simulink model "tetheredKiteModel"  (R2019a)
settings: Solver=VariableStepAuto  StartTime=0.0  StopTime=20  RelTol=1e-3
undefined symbols (not defined in the file or in its folder): magnitude
libraries: angleBtw2Vecs_ul x5, accelerationCalculator_ul x5, vrlib x4
(part 1 of 2)
settings Model: Creator=jcreed2  LastModifiedBy=jcreed2
settings DataIOCC: SaveFormat=StructureWithTime

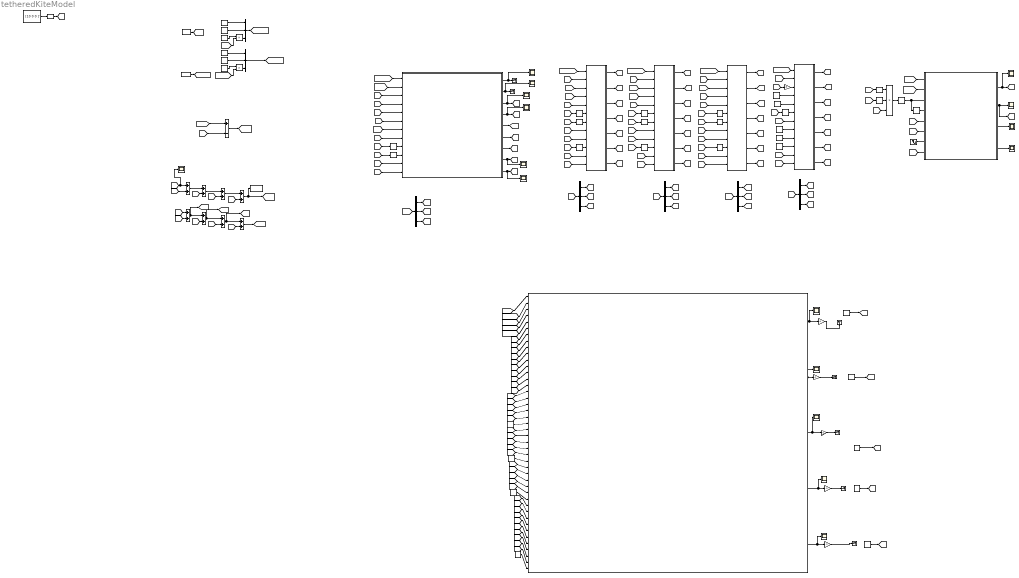
== system tetheredKiteModel ==
  note: ground position and vel.
  note: Tension Calculation
  note: Controller
  note: nodes 2-5
  note: Tether node at kite
  note: Gravity and Kite Force Calculation
  note: Kite Forces
  note: gravity force in the ground frame
  note: Force Gravity
  note: Env
  Add{,1..7} (8 alike) : Sum
  Constant : Constant  Value=[10 0 0 ]'
  Constant{1..2,5..6,10..12,15..17} (10 alike) : Constant  Value=0
  Constant13 : Constant  Value=[0,0,0]'
  Constant14 : Constant  Value=[0,0,0]'
  Constant{18..22} (5 alike) : Constant  Value=900
  Constant3 : Constant  Value=-9.81
  Constant4 : Constant  Value=20 + .5*1000*200*pi*.0005*.0005
  Constant7 : Constant  Value=-9.81
  Constant8 : Constant  Value=200
  Constant9 : Constant  Value=1000*200*pi*.0005*.0005
  Cos13 : Trigonometry  Operator=cos
  Cos14 : Trigonometry  Operator=cos
  Demux{,1..4} (5 alike) : Demux  Outputs=3
  Divide : Product  Inputs=**
  Divide1 : Product  Inputs=**
  Divide28 : Product  Inputs=***
  MATLAB Function2 : MATLAB Function  TreatAsAtomicUnit=on
  Memory{,1..13} (14 alike) : Memory
  Minus : Sum  Inputs=+-
  Multiply : Gain  Gain=.5
  Multiply{1..5} (5 alike) : Gain  Gain=-1
  Reshape : Reshape  OutputDimensionality=Column vector (2-D)
  Scope{,1..12,14..16} (16 alike) : Scope
  Sine Wave : Sin  Amplitude=60  Frequency=1/20  SampleTime=0
  Subsystem : Subsystem  mask{ky1=.1, ky=.01, kydot=.1, kalpha=0.001, rMin=-0.3491, rMax=0.3491, aMin=-0.0873, aMax=0.0873}
      mask prompts: rMin "roll min"; rMax "roll max"; aMin "aoaBar min"; aMax "aoaBar max"
  Terminator{,1..6} (7 alike) : Terminator
  To Workspace : ToWorkspace  VariableName=kitePos  SaveFormat=Timeseries  SampleTime=-1
  Vector Concatenate : Concatenate  NumInputs=3
  Vector Concatenate1 : Concatenate  NumInputs=3
  node2 : Subsystem  mask{rho=1.23, cD=1.2, lq=200, d=.001}
      mask prompts: lq "linkLength"; d "tether diameter"
  node3 : Subsystem  mask{rho=1.23, cD=1.2, lq=200, d=.001}
      mask prompts: lq "linkLength"; d "tether diameter"
  node4 : Subsystem  mask{rho=1.23, cD=1.2, lq=200, d=.001}
      mask prompts: lq "linkLength"; d "tether diameter"
  "node5 " : Subsystem  mask{rho=1.23, cD=1.2, lq=200, d=.001}
      mask prompts: lq "linkLength"; d "tether diameter"
  "tether node one (kite end of the tether) " : Subsystem  mask{cLA=4.4, S=25, rho=1.23, cD=1.2, lq=200, d=.001, cdO=.02, kO=.1}
      mask prompts: lq "linkLength"; d "tetherDiameter"; cdO "cd0"; kO "k0"
  wires:
  Constant/1 -> Reshape/1
  Reshape/1 -> [vWind]
  Constant1/1 -> Vector Concatenate/1
  Constant2/1 -> Vector Concatenate/2
  Constant3/1 -> Divide/1
  Constant4/1 -> [kiteMass]
  Divide/1 -> Vector Concatenate/3
  Vector Concatenate/1 -> [FGravKite]
  Divide1/1 -> Vector Concatenate1/3
  Constant6/1 -> Vector Concatenate1/2
  Constant5/1 -> Vector Concatenate1/1
  [tetherNodeMass] -> Divide1/2
  Constant7/1 -> Divide1/1
  Vector Concatenate1/1 -> [FGravTetherNodes]
  [FGravKite] -> "tether node one (kite end of the tether) "/1(kiteGrav)
  Constant9/1 -> [tetherNodeMass]
  [kiteMass] -> Divide/2
  [vWind] -> Minus/2
  [link1Vel] -> Minus/1  "kiteVel"
  Minus/1 -> [vRelGnd]  "vRel"
  [vRelGnd] -> Subsystem/2("vRelGnd ")
  Subsystem/1(roll) -> Scope/1, [roll]
  Subsystem/2(alpha) -> Scope3/1, [alpha]
  "tether node one (kite end of the tether) "/2("fDrag ") -> Scope12/1, Terminator/1  "fDrag"
  "tether node one (kite end of the tether) "/1("fLift ") -> Scope11/1, Terminator1/1  "fLift"
  "tether node one (kite end of the tether) "/5(fExt1) -> [fExtKite]  "fExt1"
  "tether node one (kite end of the tether) "/3(theta1) -> Scope9/1, [theta1]
  "tether node one (kite end of the tether) "/4(phi1) -> Scope10/1, [phi1]
  [theta1] -> Subsystem/5(theta)
  [phi1] -> Subsystem/6(phi)
  [vRelGnd] -> "tether node one (kite end of the tether) "/2(vRelGnd)
  [alpha] -> "tether node one (kite end of the tether) "/4(alpha)
  [roll] -> "tether node one (kite end of the tether) "/3(roll)
  [vWind] -> "tether node one (kite end of the tether) "/5(vWind)
  "tether node one (kite end of the tether) "/6("r1 ") -> [r1]
  "tether node one (kite end of the tether) "/7(r1Dot) -> [r1Dot]  "r1Dot"
  [fExtKite] -> Demux/1
  Demux/1 -> [fx1]
  Demux/2 -> [fy1]
  Demux/3 -> [fz1]
  [tetherNodeMass] -> MATLAB Function2/2(m2)
  [kiteMass] -> MATLAB Function2/1(m1)
  [tetherNodeMass] -> MATLAB Function2/3(m3)
  [tetherNodeMass] -> MATLAB Function2/4(m4)
  [tetherNodeMass] -> MATLAB Function2/5(m5)
  [phi1] -> MATLAB Function2/11(p1)
  [theta1] -> MATLAB Function2/6(t1)
  [fx1] -> MATLAB Function2/16(fx1)
  [fz1] -> MATLAB Function2/28(fz1)
  [fy1] -> MATLAB Function2/22(fy1)
  "tether node one (kite end of the tether) "/8(p1d) -> Scope14/1, [p1d]
  [p1d] -> MATLAB Function2/39(p1d)
  [t1d] -> MATLAB Function2/34(t1d)
  Constant8/1 -> MATLAB Function2/44(L)
  MATLAB Function2/3(ten3) -> Scope6/1, Multiply3/1  "ten3"
  MATLAB Function2/4(ten4) -> Scope7/1, Multiply4/1  "ten4"
  MATLAB Function2/5(ten5) -> Scope8/1, Multiply5/1  "ten5"
  [ten1] -> Memory1/1
  [FGravTetherNodes] -> node2/1(nodeGrav)
  [vWind] -> node2/2(vWind)
  [ten2] -> Memory3/1
  [ten1] -> Memory4/1
  [ten2] -> Memory2/1
  [theta1] -> node2/11(thetaq01)
  [phi1] -> node2/12(phiq01)
  [ten3] -> Memory7/1
  node2/5(rqDot) -> [r2Dot]  "r2Dot"
  node2/4("rq ") -> [r2]
  node2/3(fExtq) -> [fExt2]  "fExt2"
  node2/6(pqd) -> [p2d]
  node2/7(tqd) -> [t2d]
  node2/2(phiq) -> [phi2]
  node2/1(thetaq) -> [theta2]
  [fExt2] -> "tether node one (kite end of the tether) "/8(Fext2)
  [theta2] -> "tether node one (kite end of the tether) "/11("theta2 ")
  [phi2] -> "tether node one (kite end of the tether) "/12(phi2)
  Demux1/3 -> [fz2]
  [fExt2] -> Demux1/1
  Demux1/1 -> [fx2]
  Demux1/2 -> [fy2]
  [fx2] -> MATLAB Function2/17(fx2)
  [fy2] -> MATLAB Function2/23(fy2)
  [fz2] -> MATLAB Function2/29(fz2)
  [phi2] -> MATLAB Function2/12(p2)
  [theta2] -> MATLAB Function2/7(t2)
  [p2d] -> MATLAB Function2/40(p2d)
  [t2d] -> MATLAB Function2/35(t2d)
  [FGravTetherNodes] -> node3/1(nodeGrav)
  node3/1(thetaq) -> [theta3]
  node3/2(phiq) -> [phi3]
  node3/5(rqDot) -> [r3Dot]  "r3Dot"
  node3/7(tqd) -> [t3d]
  [ten3] -> Memory5/1
  [vWind] -> node3/2(vWind)
  [theta2] -> node3/11(thetaq01)
  [ten4] -> Memory8/1
  node3/6(pqd) -> [p3d]
  [ten2] -> Memory6/1
  node3/3(fExtq) -> [fExt3]  "fExt3"
  [phi2] -> node3/12(phiq01)
  node3/4("rq ") -> [r3]
  [theta3] -> node2/8("thetaq1 ")
  [phi3] -> node2/9(phiq1)
  [fExt3] -> node2/5(Fextq1)
  [fExt3] -> Demux2/1
  Demux2/2 -> [fy3]
  Demux2/1 -> [fx3]
  Demux2/3 -> [fz3]
  [theta3] -> MATLAB Function2/8(t3)
  [phi3] -> MATLAB Function2/13(p3)
  [fx3] -> MATLAB Function2/18(fx3)
  [fy3] -> MATLAB Function2/24(fy3)
  [fz3] -> MATLAB Function2/30(fz3)
  [t3d] -> MATLAB Function2/36(t3d)
  [p3d] -> MATLAB Function2/41(p3d)
  [p4d] -> MATLAB Function2/42(p4d)
  [p5d] -> MATLAB Function2/43(p5d)
  [t5d] -> MATLAB Function2/38(t5d)
  [t4d] -> MATLAB Function2/37(t4d)
  [fz4] -> MATLAB Function2/31(fz4)
  [fz5] -> MATLAB Function2/32(fz5)
  [fy4] -> MATLAB Function2/25(fy4)
  [fy5] -> MATLAB Function2/26(fy5)
  [fx5] -> MATLAB Function2/20(fx5)
  [fx4] -> MATLAB Function2/19(fx4)
  [phi5] -> MATLAB Function2/15(p5)
  [phi4] -> MATLAB Function2/14(p4)
  [theta4] -> MATLAB Function2/9(t4)
  [theta5] -> MATLAB Function2/10(t5)
  Demux3/2 -> [fy4]
  Demux3/3 -> [fz4]
  Demux3/1 -> [fx4]
  node4/4("rq ") -> [r4]
  [ten3] -> Memory10/1
  [phi3] -> node4/12(phiq01)
  node4/3(fExtq) -> [fExt4]  "fExt4"
  [fExt4] -> Demux3/1
  [ten4] -> Memory9/1
  [vWind] -> node4/2(vWind)
  node4/7(tqd) -> [t4d]
  node4/5(rqDot) -> [r4Dot]  "r4Dot"
  [ten5] -> Memory11/1
  [theta3] -> node4/11(thetaq01)
  node4/1(thetaq) -> [theta4]
  node4/6(pqd) -> [p4d]
  node4/2(phiq) -> [phi4]
  [FGravTetherNodes] -> node4/1(nodeGrav)
  [theta4] -> node3/8("thetaq1 ")
  [phi4] -> node3/9(phiq1)
  [fExt4] -> node3/5(Fextq1)
  [fExt5] -> node4/5(Fextq1)
  [theta5] -> node4/8("thetaq1 ")
  [phi5] -> node4/9(phiq1)
  Constant11/1 -> "node5 "/9(phiq1)
  Constant12/1 -> "node5 "/8("thetaq1 ")
  "node5 "/2(phiq) -> [phi5]
  Constant10/1 -> "node5 "/10(tenq1)
  "node5 "/1(thetaq) -> [theta5]
  "node5 "/5(rqDot) -> [r5Dot]  "r5Dot"
  "node5 "/7(tqd) -> [t5d]
  [ten4] -> "node5 "/7(tenq01)
  [theta4] -> "node5 "/11(thetaq01)
  [ten5] -> Memory12/1
  "node5 "/3(fExtq) -> [fExt5]  "fExt5"
  [FGravTetherNodes] -> "node5 "/1(nodeGrav)
  "node5 "/6(pqd) -> [p5d]
  "node5 "/4("rq ") -> [r5]
  [vWind] -> "node5 "/2(vWind)
  [phi4] -> "node5 "/12(phiq01)
  [r5] -> Scope2/1, Add/1  "node5Pos"
  [r4] -> Add/2
  Add/1 -> Add1/1  "node4Pos"
  Add1/1 -> Add2/1  "node3Pos"
  [r3] -> Add1/2
  Constant13/1 -> "node5 "/4(linkQ1VelGnd)
  [fExt5] -> Demux4/1
  Demux4/1 -> [fx5]
  Demux4/2 -> [fy5]
  Demux4/3 -> [fz5]
  [r2] -> Add2/2
  Add2/1 -> Add3/1  "node2Pos"
  [r1] -> Add3/2
  Add3/1 -> To Workspace/1, [kitePosGnd]  "kitePosGnd"
  [kitePosGnd] -> Subsystem/1("kitePosGnd ")
  [r4Dot] -> Add4/2
  Add4/1 -> [link4Vel], Add5/1  "link4Vel"
  [r1Dot] -> Add7/2
  [r5Dot] -> Add4/1
  [r2Dot] -> Add6/2
  [r3Dot] -> Add5/2
  Add5/1 -> Add6/1, [link3Vel]  "link3Vel"
  Add7/1 -> [link1Vel]
  Add6/1 -> [link2Vel], Add7/1
  Multiply/1 -> "node5 "/3("linkQVelGnd ")
  [link2Vel] -> "tether node one (kite end of the tether) "/7(link2VelGnd)  "link2Vel"
  [link3Vel] -> node2/4(linkQ1VelGnd)
  [link2Vel] -> node2/3("linkQVelGnd ")
  [link1Vel] -> "tether node one (kite end of the tether) "/6("kiteVelGnd ")
  [link3Vel] -> node3/3("linkQVelGnd ")
  [link4Vel] -> node3/4(linkQ1VelGnd)
  [link4Vel] -> node4/3("linkQVelGnd ")
  [r5Dot] -> node4/4(linkQ1VelGnd)
  Sine Wave/1 -> Subsystem/7("sineWave ")
  Memory/1 -> Subsystem/4("Tk01 ")
  Divide28/1 -> Memory13/1
  Cos13/1 -> Divide28/1
  [ten1] -> Divide28/3
  [theta1] -> Cos13/1
  Cos14/1 -> Divide28/2
  [phi1] -> Cos14/1
  Constant14/1 -> "node5 "/5(Fextq1)
  Constant15/1 -> MATLAB Function2/21(fx6)
  Constant17/1 -> MATLAB Function2/33(fz6)
  Constant16/1 -> MATLAB Function2/27(fy6)
  Memory1/1 -> "tether node one (kite end of the tether) "/9("ten1 ")
  Memory2/1 -> "tether node one (kite end of the tether) "/10(ten2)
  Memory4/1 -> node2/7(tenq01)
  Memory3/1 -> node2/6("tenq ")
  Memory5/1 -> node3/6("tenq ")
  Memory6/1 -> node3/7(tenq01)
  Memory7/1 -> node2/10(tenq1)
  Memory8/1 -> node3/10(tenq1)
  Memory9/1 -> node4/6("tenq ")
  Memory10/1 -> node4/7(tenq01)
  Memory11/1 -> node4/10(tenq1)
  Memory12/1 -> "node5 "/6("tenq ")
  Memory13/1 -> Memory/1, Subsystem/3("Tc ")
  [link1Vel] -> Subsystem/8("kiteVelGnd ")
  Subsystem/3(error) -> Scope1/1
  [r5Dot] -> Multiply/1
  MATLAB Function2/1(ten1) -> Scope4/1, Multiply1/1  "ten"
  MATLAB Function2/2(ten2) -> Scope5/1, Multiply2/1  "ten2"
  "tether node one (kite end of the tether) "/9(t1d) -> Scope15/1, [t1d]
  Multiply1/1 -> Terminator2/1
  Multiply3/1 -> Terminator4/1
  Multiply5/1 -> Terminator6/1
  Subsystem/4(tenError) -> Scope16/1
  Constant18/1 -> [ten1]
  Constant19/1 -> [ten2]
  Multiply2/1 -> Terminator3/1
  Constant20/1 -> [ten3]
  Constant21/1 -> [ten4]
  Multiply4/1 -> Terminator5/1
  Constant22/1 -> [ten5]

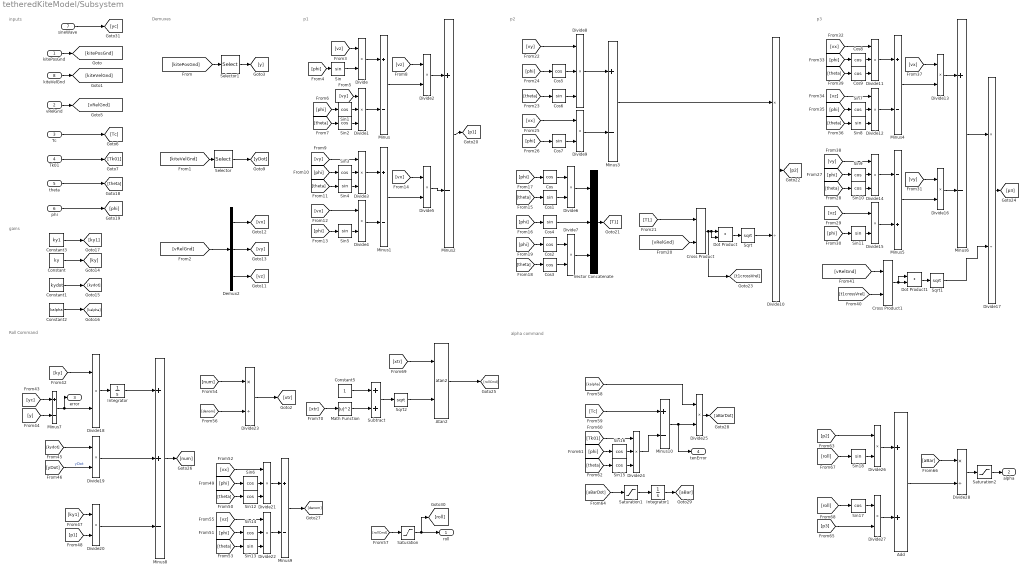
== system tetheredKiteModel/Subsystem ==
  note: alpha command
  note: Roll Command
  note: p2
  note: p1
  note: gains
  note: Demuxes
  note: inputs
  note: p3
  "kitePosGnd " : Inport
  "vRelGnd " : Inport  Port=2
  "Tc " : Inport  Port=3
  "Tk01 " : Inport  Port=4
  theta : Inport  Port=5
  phi : Inport  Port=6
  "sineWave " : Inport  Port=7
  "kiteVelGnd " : Inport  Port=8
  Add : Sum
  Atan2 : Trigonometry  Operator=atan2
  Constant : Constant  Value=ky
  Constant1 : Constant  Value=kydot
  Constant2 : Constant  Value=kalpha
  Constant3 : Constant  Value=ky1
  Constant5 : Constant
  Cos{,2..3,5,8..9} (6 alike) : Trigonometry  Operator=cos
  Cos{1,4,6..7} (4 alike) : Trigonometry
  Cross Product : vrlib/Utilities/Cross Product
      settings: SourceProductName=Simulink
  Cross Product1 : vrlib/Utilities/Cross Product
      settings: SourceProductName=Simulink
  Demux2 : Demux  Outputs=3
  Divide{,2,4..7,9,13,15..16,18..20,25..27} (16 alike) : Product  Inputs=**
  Divide{1,3,8,11..12,14,21..22,24} (9 alike) : Product  Inputs=***
  Divide{10,17,23,28} (4 alike) : Product  Inputs=*/
  Dot Product : DotProduct  InputSameDT=on  OutDataTypeStr=Inherit: Inherit via internal rule
  Dot Product1 : DotProduct  InputSameDT=on  OutDataTypeStr=Inherit: Inherit via internal rule
  Integrator : Integrator
  Integrator1 : Integrator
  Math Function : Math  Operator=magnitude^2  SaturateOnIntegerOverflow=on
  Minus{,1..4,6..7,9..10} (9 alike) : Sum  Inputs=+-
  Minus5 : Sum  Inputs=-+
  Minus8 : Sum  Inputs=++-
  Saturation : Saturate  UpperLimit=rMax  LowerLimit=rMin
  Saturation1 : Saturate  UpperLimit=aMax  LowerLimit=aMin
  Saturation2 : Saturate  UpperLimit=0.0349*4  LowerLimit=0.0349
  Selector : Selector  InputPortWidth=3  IndexOptions=Index vector (dialog)  Indices=2  OutputSizes=1
  Selector1 : Selector  InputPortWidth=3  IndexOptions=Index vector (dialog)  Indices=2  OutputSizes=1
  Sin{,4..5,8,11,13,18} (7 alike) : Trigonometry
  Sin{1..3,6..7,9..10,12,14..17} (12 alike) : Trigonometry  Operator=cos
  Sqrt : Sqrt  SaturateOnIntegerOverflow=on
  Sqrt1 : Sqrt  SaturateOnIntegerOverflow=on
  Sqrt2 : Sqrt  SaturateOnIntegerOverflow=on
  Subtract : Sum
  Vector Concatenate : Concatenate  NumInputs=3
  roll : Outport
  alpha : Outport  Port=2
  error : Outport  Port=3
  tenError : Outport  Port=4
  wires:
  "kitePosGnd "/1 -> [kitePosGnd]
  "kiteVelGnd "/1 -> [kiteVelGnd]
  "vRelGnd "/1 -> [vRelGnd]
  "Tc "/1 -> [Tc]
  "Tk01 "/1 -> [Tk01]
  [kiteVelGnd] -> Selector/1
  Selector/1 -> [yDot]
  [vRelGnd] -> Demux2/1
  Demux2/1 -> [vx]
  Demux2/2 -> [vy]
  Demux2/3 -> [vz]
  Constant/1 -> [ky]
  Constant1/1 -> [kydot]
  Constant2/1 -> [kalpha]
  Constant3/1 -> [ky1]
  theta/1 -> [theta]
  phi/1 -> [phi]
  [vz] -> Divide/1
  Sin/1 -> Divide/2
  [phi] -> Sin/1
  [vy] -> Divide1/1
  Sin1/1 -> Divide1/2
  Sin2/1 -> Divide1/3
  [phi] -> Sin1/1
  [theta] -> Sin2/1
  Divide/1 -> Minus/1
  Divide1/1 -> Minus/2
  Minus/1 -> Divide2/2
  [vz] -> Divide2/1
  Sin3/1 -> Divide3/2
  [phi] -> Sin3/1
  [vy] -> Divide3/1
  [theta] -> Sin4/1
  Sin4/1 -> Divide3/3
  Sin5/1 -> Divide4/2
  [phi] -> Sin5/1
  [vx] -> Divide4/1
  Divide3/1 -> Minus1/1
  Divide4/1 -> Minus1/2
  Minus1/1 -> Divide5/2
  [vx] -> Divide5/1
  Divide2/1 -> Minus2/1
  Divide5/1 -> Minus2/2
  Minus2/1 -> [p1]
  Cos/1 -> Divide6/1
  Divide6/1 -> Vector Concatenate/1
  Cos1/1 -> Divide6/2
  Divide7/1 -> Vector Concatenate/3
  Cos2/1 -> Divide7/1
  Cos3/1 -> Divide7/2
  Cos4/1 -> Vector Concatenate/2
  [phi] -> Cos4/1
  [theta] -> Cos1/1
  [phi] -> Cos/1
  [theta] -> Cos3/1
  [phi] -> Cos2/1
  Vector Concatenate/1 -> [T1]
  [vRelGnd] -> Cross Product/2
  [T1] -> Cross Product/1
  Cross Product/1 -> [t1crossVrel], Dot Product/2, Dot Product/1
  Dot Product/1 -> Sqrt/1
  Cos5/1 -> Divide8/2
  Cos6/1 -> Divide8/3
  [theta] -> Cos6/1
  [phi] -> Cos5/1
  [vy] -> Divide8/1
  Divide8/1 -> Minus3/1
  [vx] -> Divide9/1
  Cos7/1 -> Divide9/2
  [phi] -> Cos7/1
  Divide9/1 -> Minus3/2
  Minus3/1 -> Divide10/1
  Divide10/1 -> [p2]
  [theta] -> Sin8/1
  Divide12/1 -> Minus4/2
  Divide11/1 -> Minus4/1
  [vz] -> Divide12/1
  [phi] -> Sin7/1
  Sin10/1 -> Divide14/3
  [phi] -> Sin9/1
  [vy] -> Divide14/1
  [vy] -> Divide16/1
  Divide16/1 -> Minus6/2
  [vx] -> Divide13/1
  Sin8/1 -> Divide12/3
  [phi] -> Cos8/1
  Sin7/1 -> Divide12/2
  Minus6/1 -> Divide17/1
  Sin11/1 -> Divide15/2
  Divide13/1 -> Minus6/1
  Divide14/1 -> Minus5/1
  Minus5/1 -> Divide16/2
  Divide15/1 -> Minus5/2
  Minus4/1 -> Divide13/2
  [vz] -> Divide15/1
  Sin9/1 -> Divide14/2
  [phi] -> Sin11/1
  [theta] -> Sin10/1
  [vx] -> Divide11/1
  Cos8/1 -> Divide11/2
  Cos9/1 -> Divide11/3
  [theta] -> Cos9/1
  [t1crossVrel] -> Cross Product1/2
  [vRelGnd] -> Cross Product1/1
  Cross Product1/1 -> Dot Product1/1, Dot Product1/2
  Dot Product1/1 -> Sqrt1/1
  Sqrt1/1 -> Divide17/2
  Divide17/1 -> [p3]
  [yc] -> Minus7/1
  [y] -> Minus7/2
  Minus7/1 -> Divide18/2, error/1
  [ky] -> Divide18/1
  Divide18/1 -> Integrator/1
  [kydot] -> Divide19/1
  [yDot] -> Divide19/2  "yDot"
  Integrator/1 -> Minus8/1
  Divide19/1 -> Minus8/2
  [ky1] -> Divide20/1
  [p1] -> Divide20/2
  Divide20/1 -> Minus8/3
  Minus8/1 -> [num]
  Sin12/1 -> Divide21/3
  [phi] -> Sin6/1
  [vx] -> Divide21/1
  Sin6/1 -> Divide21/2
  [theta] -> Sin12/1
  Divide21/1 -> Minus9/1
  [theta] -> Sin13/1
  Sin14/1 -> Divide22/2
  Sin13/1 -> Divide22/3
  [vz] -> Divide22/1
  [phi] -> Sin14/1
  Divide22/1 -> Minus9/2
  Minus9/1 -> [denom]
  Divide23/1 -> [xtr]
  [num] -> Divide23/1
  [denom] -> Divide23/2
  [rollCmd] -> Saturation/1
  Saturation/1 -> [roll], roll/1
  Sin16/1 -> Divide24/2
  Sin15/1 -> Divide24/3
  [phi] -> Sin16/1
  [Tk01] -> Divide24/1
  [theta] -> Sin15/1
  [Tc] -> Minus10/1
  Divide24/1 -> Minus10/2
  Minus10/1 -> tenError/1, Divide25/2
  [kalpha] -> Divide25/1
  Divide25/1 -> [aBarDot]
  [aBarDot] -> Saturation1/1
  Saturation1/1 -> Integrator1/1
  Integrator1/1 -> [aBar]
  [roll] -> Sin18/1
  [roll] -> Sin17/1
  Sin18/1 -> Divide26/2
  [p2] -> Divide26/1
  Sin17/1 -> Divide27/1
  [p3] -> Divide27/2
  Divide26/1 -> Add/1
  Divide27/1 -> Add/2
  [aBar] -> Divide28/1
  Add/1 -> Divide28/2
  Divide28/1 -> Saturation2/1
  Sqrt/1 -> Divide10/2
  "sineWave "/1 -> [yc]
  Saturation2/1 -> alpha/1
  [kitePosGnd] -> Selector1/1
  Selector1/1 -> [y]
  [xtr] -> Atan2/1
  Constant5/1 -> Subtract/1
  [xtr] -> Math Function/1
  Math Function/1 -> Subtract/2
  Subtract/1 -> Sqrt2/1
  Sqrt2/1 -> Atan2/2
  Atan2/1 -> [rollCmd]

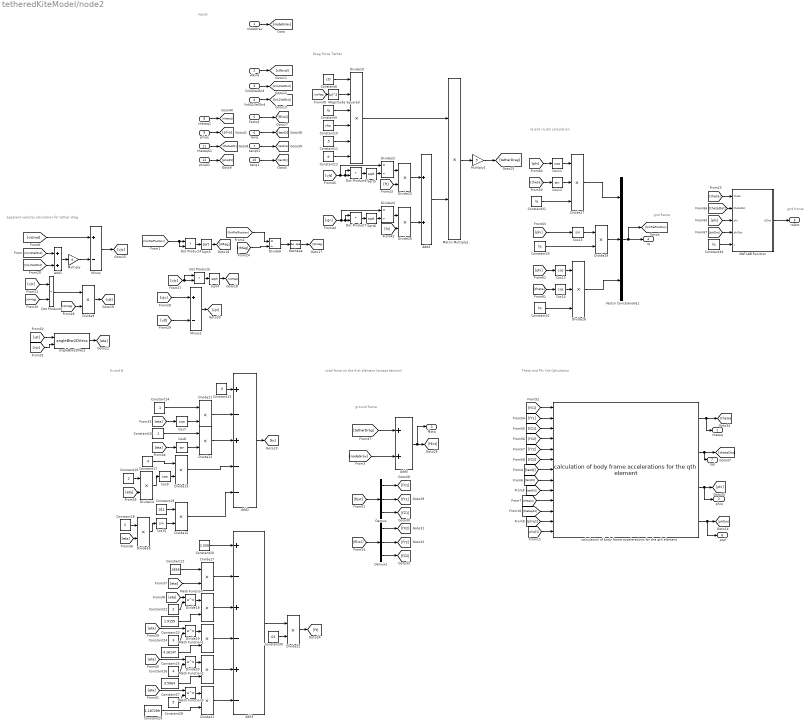
== system tetheredKiteModel/node2 ==
  note: gnd frame
  note: fn and ft
  note: gnd frame
  note: inputs
  note: apparent velocity calculation for tether drag
  note: ground frame
  note: rq and rq dot calculation
  note: Theta and Phi link Calculation
  note: total force on the first element
      |  (except tension)
  note: Drag Force Tether
  nodeGrav : Inport
  vWind : Inport  Port=2
  "linkQVelGnd " : Inport  Port=3
  linkQ1VelGnd : Inport  Port=4
  Fextq1 : Inport  Port=5
  "tenq " : Inport  Port=6
  tenq01 : Inport  Port=7
  "thetaq1 " : Inport  Port=8
  phiq1 : Inport  Port=9
  tenq1 : Inport  Port=10
  thetaq01 : Inport  Port=11
  phiq01 : Inport  Port=12
  Add1 : Sum
  Add2 : Sum  Inputs=+-+--
  Add3 : Sum  Inputs=+-+-+-
  Add4 : Sum
  Add5 : Sum
  Constant10 : Constant  Value=rho
  Constant11 : Constant  Value=.5
  Constant12 : Constant  Value=d
  Constant13 : Constant  Value=.5
  Constant14 : Constant  Value=.1
  Constant15 : Constant  Value=.1
  Constant16 : Constant  Value=2
  Constant17 : Constant  Value=.4
  Constant18 : Constant  Value=2
  Constant19 : Constant  Value=.011
  Constant20 : Constant  Value=2.008
  Constant21 : Constant  Value=.3858
  Constant22 : Constant  Value=2
  Constant23 : Constant  Value=1.9159
  Constant24 : Constant  Value=3
  Constant25 : Constant  Value=4.16147
  Constant26 : Constant  Value=4
  Constant27 : Constant  Value=3.5064
  Constant28 : Constant  Value=5
  Constant29 : Constant  Value=1.187299
  Constant30 : Constant  Value=.01
  Constant{9,31..34} (5 alike) : Constant  Value=lq
  Constant8 : Constant  Value=cD
  Cos{8,10,12,15} (4 alike) : Trigonometry
  Cos{7,9,11,13..14} (5 alike) : Trigonometry  Operator=cos
  Demux : Demux  Outputs=3
  Demux1 : Demux  Outputs=3
  Divide10 : Product  Inputs=******
  Divide{9,11..22,25..26,29} (16 alike) : Product  Inputs=**
  Divide23 : Product  Inputs=*/
  Divide24 : Product  Inputs=*/
  Divide27 : Product  Inputs=***
  Divide28 : Product  Inputs=***
  Divide8 : Product  Inputs=*/
  Dot Product{3..7} (5 alike) : DotProduct  InputSameDT=on  OutDataTypeStr=Inherit: Inherit via internal rule
  MATLAB Function : MATLAB Function  TreatAsAtomicUnit=on
  Magnitude Squared : Math  Operator=magnitude^2  SaturateOnIntegerOverflow=on
  Math Function{,1..3} (4 alike) : Math  Operator=pow  SaturateOnIntegerOverflow=on
  Matrix Multiply2 : Product
  Minus : Sum  Inputs=+-
  Minus1 : Sum  Inputs=+-
  Multiply : Gain  Gain=.5
  Multiply1 : Gain  Gain=.5
  Reshape : Reshape  OutputDimensionality=Column vector (2-D)
  Sqrt{3..6} (4 alike) : Sqrt  SaturateOnIntegerOverflow=on
  Vector Concatenate1 : Concatenate  NumInputs=3
  angleBtw2DVecs : angleBtw2Vecs_ul/angleBtw2DVecs  SystemSampleTime=-1
  calculation of body frame accelerations for the qth element : accelerationCalculator_ul/calculation of body frame accelerations for the qth element  mj=1000*200*pi*.0005*.0005  mj1=1000*200*pi*.0005*.0005  L=200
  thetaq : Outport
  phiq : Outport  Port=2
  fExtq : Outport  Port=3
  "rq " : Outport  Port=4
  rqDot : Outport  Port=5
  pqd : Outport  Port=6
  tqd : Outport  Port=7
  wires:
  Cos14/1 -> Divide28/2
  Constant32/1 -> Divide28/3
  Cos15/1 -> Divide29/1
  Constant34/1 -> MATLAB Function/5(L)
  Demux/3 -> [fZ1]
  Divide16/1 -> Cos10/1
  Cos10/1 -> Divide15/2
  Constant18/1 -> Divide16/1
  Divide21/1 -> Add3/6
  Constant21/1 -> Divide17/1
  [fZ1] -> calculation of body frame accelerations for the qth element/3
  tenq01/1 -> [tenQ01]
  [phi] -> Cos15/1
  MATLAB Function/1(r1Dot) -> rqDot/1
  [vJc] -> angleBtw2DVecs/2
  Magnitude Squared/1 -> Divide10/2
  [phi] -> Cos11/1
  [fExt] -> Demux/1
  [phiq01] -> calculation of body frame accelerations for the qth element/13
  Demux1/2 -> [fY2]
  Constant14/1 -> Divide11/1
  Demux1/1 -> [fX2]
  [eta] -> Divide17/2
  [phi] -> MATLAB Function/3(phi)
  Divide22/1 -> [ft]
  Divide15/1 -> Add2/5
  Constant11/1 -> Divide10/5
  Constant12/1 -> Divide10/6
  Divide19/1 -> Add3/4
  Cos12/1 -> Divide27/2
  [tetherDrag] -> Add5/1
  [thetaDot] -> MATLAB Function/2(thetaDot)
  [vJc] -> Dot Product5/1, Dot Product5/2
  [rMag] -> Divide8/2
  [eta] -> Cos8/1
  Constant15/1 -> Divide12/1
  Sqrt4/1 -> [vJcMag]
  Add3/1 -> Divide22/1
  Divide27/1 -> Vector Concatenate1/1
  Cos13/1 -> Divide28/1
  Sqrt3/1 -> [rMag]
  Add4/1 -> Matrix Multiply2/2
  Cos7/1 -> Divide11/2
  Multiply/1 -> Minus/2
  Vector Concatenate1/1 -> [linkRelPosition], "rq "/1
  Divide11/1 -> Add2/2
  Dot Product5/1 -> Sqrt4/1
  [vJcMag] -> Magnitude Squared/1
  Minus/1 -> [vJc]
  [theta] -> Cos14/1
  Constant33/1 -> Divide29/2
  [theta] -> MATLAB Function/1(theta)
  [rDrMag] -> Divide9/2
  Minus1/1 -> [vJn]
  Divide8/1 -> Reshape/1
  Dot Product3/1 -> Divide9/1
  [vJt] -> angleBtw2DVecs/1
  nodeGrav/1 -> [nodeGrav]
  [fX2] -> calculation of body frame accelerations for the qth element/4
  Constant23/1 -> Divide18/2
  [fY2] -> calculation of body frame accelerations for the qth element/5
  [fZ2] -> calculation of body frame accelerations for the qth element/6
  Divide29/1 -> Vector Concatenate1/2
  [vJc] -> Dot Product3/1
  Divide18/1 -> Add3/3
  [phi] -> Cos13/1
  Constant10/1 -> Divide10/4
  Constant8/1 -> Divide10/1
  [eta] -> Cos7/1
  Constant9/1 -> Divide10/3
  Divide17/1 -> Add3/2
  Dot Product4/1 -> Sqrt3/1
  Constant19/1 -> Divide15/1
  Add2/1 -> [fn]
  [vJt] -> Divide23/1, Dot Product6/1, Dot Product6/2
  Add5/1 -> fExtq/1, [fExt]
  Constant13/1 -> Add2/1
  Dot Product6/1 -> Sqrt5/1
  Constant26/1 -> Math Function2/2
  [vWind] -> Minus/1
  [vJc] -> Minus1/1
  Math Function2/1 -> Divide20/1
  [eta] -> Math Function2/1
  Constant27/1 -> Divide20/2
  Fextq1/1 -> [fExt2]
  vWind/1 -> [vWind]
  [rDrMag] -> Dot Product3/2
  [phiDot] -> MATLAB Function/4(phiDot)
  Demux/2 -> [fY1]
  Divide23/1 -> Divide25/1
  Divide26/1 -> Add4/2
  [eta] -> Divide16/2
  Constant30/1 -> Divide22/2
  Divide25/1 -> Add4/1
  Divide9/1 -> [vJt]
  Constant24/1 -> Math Function1/2
  Math Function1/1 -> Divide19/1
  Sqrt6/1 -> Divide24/2
  Demux1/3 -> [fZ2]
  Add1/1 -> Multiply/1
  [link2VelGnd] -> Add1/2
  [fX1] -> calculation of body frame accelerations for the qth element/1
  [ft] -> Divide25/2
  Constant20/1 -> Add3/1
  Divide20/1 -> Add3/5
  [thetaq1] -> calculation of body frame accelerations for the qth element/10
  "thetaq1 "/1 -> [thetaq1]
  [linkRelPosition] -> Dot Product4/2, Dot Product4/1
  [tenQ01] -> calculation of body frame accelerations for the qth element/9
  phiq1/1 -> [phiq1]
  [eta] -> Math Function3/1
  Cos8/1 -> Divide12/2
  Constant25/1 -> Divide19/2
  angleBtw2DVecs/1 -> [eta]
  Constant28/1 -> Math Function3/2
  [eta] -> Divide14/2
  Math Function3/1 -> Divide21/1
  linkQ1VelGnd/1 -> [link2VelGnd]
  Constant29/1 -> Divide21/2
  Divide24/1 -> Divide26/1
  [vJn] -> Divide24/1, Dot Product7/1, Dot Product7/2
  [tenQ] -> calculation of body frame accelerations for the qth element/7
  Constant16/1 -> Divide14/1
  Demux/1 -> [fX1]
  [eta] -> Math Function/1
  Constant17/1 -> Divide13/1
  [vJt] -> Minus1/2
  [linkRelPosition] -> Divide8/1
  Divide10/1 -> Matrix Multiply2/1
  [eta] -> Math Function1/1
  Matrix Multiply2/1 -> Multiply1/1
  Divide28/1 -> Vector Concatenate1/3
  [fY1] -> calculation of body frame accelerations for the qth element/2
  "linkQVelGnd "/1 -> [linkQVelGnd]
  [theta] -> Cos12/1
  Constant31/1 -> Divide27/3
  Sqrt5/1 -> Divide23/2
  [fn] -> Divide26/2
  Math Function/1 -> Divide18/1
  Divide13/1 -> Add2/4
  "tenq "/1 -> [tenQ]
  [nodeGrav] -> Add5/2
  Divide14/1 -> Cos9/1
  Constant22/1 -> Math Function/2
  Divide12/1 -> Add2/3
  [thetaq01] -> calculation of body frame accelerations for the qth element/11
  Multiply1/1 -> [tetherDrag]
  [tenQ1] -> calculation of body frame accelerations for the qth element/8
  Dot Product7/1 -> Sqrt6/1
  Cos11/1 -> Divide27/1
  [fExt2] -> Demux1/1
  [linkQVelGnd] -> Add1/1
  Cos9/1 -> Divide13/2
  tenq1/1 -> [tenQ1]
  thetaq01/1 -> [thetaq01]
  phiq01/1 -> [phiq01]
  [phiq1] -> calculation of body frame accelerations for the qth element/12
  Reshape/1 -> [rDrMag]
  calculation of body frame accelerations for the qth element/1 -> thetaq/1, [theta]
  calculation of body frame accelerations for the qth element/2 -> tqd/1, [thetaDot]
  calculation of body frame accelerations for the qth element/3 -> phiq/1, [phi]
  calculation of body frame accelerations for the qth element/4 -> pqd/1, [phiDot]

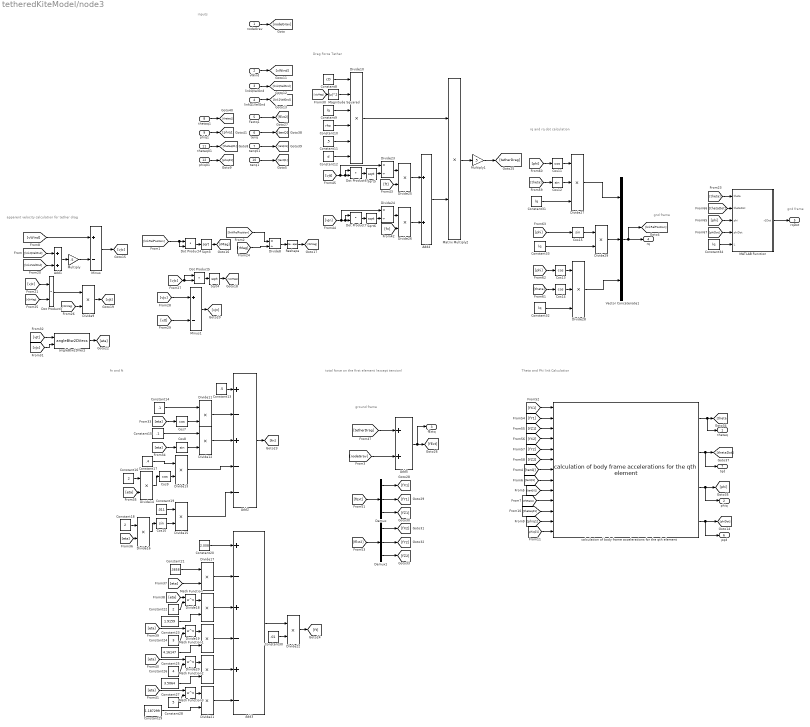
== system tetheredKiteModel/node3 ==
  note: gnd frame
  note: fn and ft
  note: gnd frame
  note: inputs
  note: apparent velocity calculation for tether drag
  note: ground frame
  note: rq and rq dot calculation
  note: Theta and Phi link Calculation
  note: total force on the first element
      |  (except tension)
  note: Drag Force Tether
  nodeGrav : Inport
  vWind : Inport  Port=2
  "linkQVelGnd " : Inport  Port=3
  linkQ1VelGnd : Inport  Port=4
  Fextq1 : Inport  Port=5
  "tenq " : Inport  Port=6
  tenq01 : Inport  Port=7
  "thetaq1 " : Inport  Port=8
  phiq1 : Inport  Port=9
  tenq1 : Inport  Port=10
  thetaq01 : Inport  Port=11
  phiq01 : Inport  Port=12
  Add1 : Sum
  Add2 : Sum  Inputs=+-+--
  Add3 : Sum  Inputs=+-+-+-
  Add4 : Sum
  Add5 : Sum
  Constant10 : Constant  Value=rho
  Constant11 : Constant  Value=.5
  Constant12 : Constant  Value=d
  Constant13 : Constant  Value=.5
  Constant14 : Constant  Value=.1
  Constant15 : Constant  Value=.1
  Constant16 : Constant  Value=2
  Constant17 : Constant  Value=.4
  Constant18 : Constant  Value=2
  Constant19 : Constant  Value=.011
  Constant20 : Constant  Value=2.008
  Constant21 : Constant  Value=.3858
  Constant22 : Constant  Value=2
  Constant23 : Constant  Value=1.9159
  Constant24 : Constant  Value=3
  Constant25 : Constant  Value=4.16147
  Constant26 : Constant  Value=4
  Constant27 : Constant  Value=3.5064
  Constant28 : Constant  Value=5
  Constant29 : Constant  Value=1.187299
  Constant30 : Constant  Value=.01
  Constant{9,31..34} (5 alike) : Constant  Value=lq
  Constant8 : Constant  Value=cD
  Cos{8,10,12,15} (4 alike) : Trigonometry
  Cos{7,9,11,13..14} (5 alike) : Trigonometry  Operator=cos
  Demux : Demux  Outputs=3
  Demux1 : Demux  Outputs=3
  Divide10 : Product  Inputs=******
  Divide{9,11..22,25..26,29} (16 alike) : Product  Inputs=**
  Divide23 : Product  Inputs=*/
  Divide24 : Product  Inputs=*/
  Divide27 : Product  Inputs=***
  Divide28 : Product  Inputs=***
  Divide8 : Product  Inputs=*/
  Dot Product{3..7} (5 alike) : DotProduct  InputSameDT=on  OutDataTypeStr=Inherit: Inherit via internal rule
  MATLAB Function : MATLAB Function  TreatAsAtomicUnit=on
  Magnitude Squared : Math  Operator=magnitude^2  SaturateOnIntegerOverflow=on
  Math Function{,1..3} (4 alike) : Math  Operator=pow  SaturateOnIntegerOverflow=on
  Matrix Multiply2 : Product
  Minus : Sum  Inputs=+-
  Minus1 : Sum  Inputs=+-
  Multiply : Gain  Gain=.5
  Multiply1 : Gain  Gain=.5
  Reshape : Reshape  OutputDimensionality=Column vector (2-D)
  Sqrt{3..6} (4 alike) : Sqrt  SaturateOnIntegerOverflow=on
  Vector Concatenate1 : Concatenate  NumInputs=3
  angleBtw2DVecs : angleBtw2Vecs_ul/angleBtw2DVecs  SystemSampleTime=-1
  calculation of body frame accelerations for the qth element : accelerationCalculator_ul/calculation of body frame accelerations for the qth element  mj=1000*200*pi*.0005*.0005  mj1=1000*200*pi*.0005*.0005  L=200
  thetaq : Outport
  phiq : Outport  Port=2
  fExtq : Outport  Port=3
  "rq " : Outport  Port=4
  rqDot : Outport  Port=5
  pqd : Outport  Port=6
  tqd : Outport  Port=7
  wires:
  Cos14/1 -> Divide28/2
  Constant32/1 -> Divide28/3
  Cos15/1 -> Divide29/1
  Constant34/1 -> MATLAB Function/5(L)
  Demux/3 -> [fZ1]
  Divide16/1 -> Cos10/1
  Cos10/1 -> Divide15/2
  Constant18/1 -> Divide16/1
  Divide21/1 -> Add3/6
  Constant21/1 -> Divide17/1
  [fZ1] -> calculation of body frame accelerations for the qth element/3
  tenq01/1 -> [tenQ01]
  [phi] -> Cos15/1
  MATLAB Function/1(r1Dot) -> rqDot/1
  [vJc] -> angleBtw2DVecs/2
  Magnitude Squared/1 -> Divide10/2
  [phi] -> Cos11/1
  [fExt] -> Demux/1
  [phiq01] -> calculation of body frame accelerations for the qth element/13
  Demux1/2 -> [fY2]
  Constant14/1 -> Divide11/1
  Demux1/1 -> [fX2]
  [eta] -> Divide17/2
  [phi] -> MATLAB Function/3(phi)
  Divide22/1 -> [ft]
  Divide15/1 -> Add2/5
  Constant11/1 -> Divide10/5
  Constant12/1 -> Divide10/6
  Divide19/1 -> Add3/4
  Cos12/1 -> Divide27/2
  [tetherDrag] -> Add5/1
  [thetaDot] -> MATLAB Function/2(thetaDot)
  [vJc] -> Dot Product5/1, Dot Product5/2
  [rMag] -> Divide8/2
  [eta] -> Cos8/1
  Constant15/1 -> Divide12/1
  Sqrt4/1 -> [vJcMag]
  Add3/1 -> Divide22/1
  Divide27/1 -> Vector Concatenate1/1
  Cos13/1 -> Divide28/1
  Sqrt3/1 -> [rMag]
  Add4/1 -> Matrix Multiply2/2
  Cos7/1 -> Divide11/2
  Multiply/1 -> Minus/2
  Vector Concatenate1/1 -> [linkRelPosition], "rq "/1
  Divide11/1 -> Add2/2
  Dot Product5/1 -> Sqrt4/1
  [vJcMag] -> Magnitude Squared/1
  Minus/1 -> [vJc]
  [theta] -> Cos14/1
  Constant33/1 -> Divide29/2
  [theta] -> MATLAB Function/1(theta)
  [rDrMag] -> Divide9/2
  Minus1/1 -> [vJn]
  Divide8/1 -> Reshape/1
  Dot Product3/1 -> Divide9/1
  [vJt] -> angleBtw2DVecs/1
  nodeGrav/1 -> [nodeGrav]
  [fX2] -> calculation of body frame accelerations for the qth element/4
  Constant23/1 -> Divide18/2
  [fY2] -> calculation of body frame accelerations for the qth element/5
  [fZ2] -> calculation of body frame accelerations for the qth element/6
  Divide29/1 -> Vector Concatenate1/2
  [vJc] -> Dot Product3/1
  Divide18/1 -> Add3/3
  [phi] -> Cos13/1
  Constant10/1 -> Divide10/4
  Constant8/1 -> Divide10/1
  [eta] -> Cos7/1
  Constant9/1 -> Divide10/3
  Divide17/1 -> Add3/2
  Dot Product4/1 -> Sqrt3/1
  Constant19/1 -> Divide15/1
  Add2/1 -> [fn]
  [vJt] -> Divide23/1, Dot Product6/1, Dot Product6/2
  Add5/1 -> fExtq/1, [fExt]
  Constant13/1 -> Add2/1
  Dot Product6/1 -> Sqrt5/1
  Constant26/1 -> Math Function2/2
  [vWind] -> Minus/1
  [vJc] -> Minus1/1
  Math Function2/1 -> Divide20/1
  [eta] -> Math Function2/1
  Constant27/1 -> Divide20/2
  Fextq1/1 -> [fExt2]
  vWind/1 -> [vWind]
  [rDrMag] -> Dot Product3/2
  [phiDot] -> MATLAB Function/4(phiDot)
  Demux/2 -> [fY1]
  Divide23/1 -> Divide25/1
  Divide26/1 -> Add4/2
  [eta] -> Divide16/2
  Constant30/1 -> Divide22/2
  Divide25/1 -> Add4/1
  Divide9/1 -> [vJt]
  Constant24/1 -> Math Function1/2
  Math Function1/1 -> Divide19/1
  Sqrt6/1 -> Divide24/2
  Demux1/3 -> [fZ2]
  Add1/1 -> Multiply/1
  [link2VelGnd] -> Add1/2
  [fX1] -> calculation of body frame accelerations for the qth element/1
  [ft] -> Divide25/2
  Constant20/1 -> Add3/1
  Divide20/1 -> Add3/5
  [thetaq1] -> calculation of body frame accelerations for the qth element/10
  "thetaq1 "/1 -> [thetaq1]
  [linkRelPosition] -> Dot Product4/2, Dot Product4/1
  [tenQ01] -> calculation of body frame accelerations for the qth element/9
  phiq1/1 -> [phiq1]
  [eta] -> Math Function3/1
  Cos8/1 -> Divide12/2
  Constant25/1 -> Divide19/2
  angleBtw2DVecs/1 -> [eta]
  Constant28/1 -> Math Function3/2
  [eta] -> Divide14/2
  Math Function3/1 -> Divide21/1
  linkQ1VelGnd/1 -> [link2VelGnd]
  Constant29/1 -> Divide21/2
  Divide24/1 -> Divide26/1
  [vJn] -> Divide24/1, Dot Product7/1, Dot Product7/2
  [tenQ] -> calculation of body frame accelerations for the qth element/7
  Constant16/1 -> Divide14/1
  Demux/1 -> [fX1]
  [eta] -> Math Function/1
  Constant17/1 -> Divide13/1
  [vJt] -> Minus1/2
  [linkRelPosition] -> Divide8/1
  Divide10/1 -> Matrix Multiply2/1
  [eta] -> Math Function1/1
  Matrix Multiply2/1 -> Multiply1/1
  Divide28/1 -> Vector Concatenate1/3
  [fY1] -> calculation of body frame accelerations for the qth element/2
  "linkQVelGnd "/1 -> [linkQVelGnd]
  [theta] -> Cos12/1
  Constant31/1 -> Divide27/3
  Sqrt5/1 -> Divide23/2
  [fn] -> Divide26/2
  Math Function/1 -> Divide18/1
  Divide13/1 -> Add2/4
  "tenq "/1 -> [tenQ]
  [nodeGrav] -> Add5/2
  Divide14/1 -> Cos9/1
  Constant22/1 -> Math Function/2
  Divide12/1 -> Add2/3
  [thetaq01] -> calculation of body frame accelerations for the qth element/11
  Multiply1/1 -> [tetherDrag]
  [tenQ1] -> calculation of body frame accelerations for the qth element/8
  Dot Product7/1 -> Sqrt6/1
  Cos11/1 -> Divide27/1
  [fExt2] -> Demux1/1
  [linkQVelGnd] -> Add1/1
  Cos9/1 -> Divide13/2
  tenq1/1 -> [tenQ1]
  thetaq01/1 -> [thetaq01]
  phiq01/1 -> [phiq01]
  [phiq1] -> calculation of body frame accelerations for the qth element/12
  Reshape/1 -> [rDrMag]
  calculation of body frame accelerations for the qth element/4 -> pqd/1, [phiDot]
  calculation of body frame accelerations for the qth element/1 -> thetaq/1, [theta]
  calculation of body frame accelerations for the qth element/2 -> tqd/1, [thetaDot]
  calculation of body frame accelerations for the qth element/3 -> phiq/1, [phi]

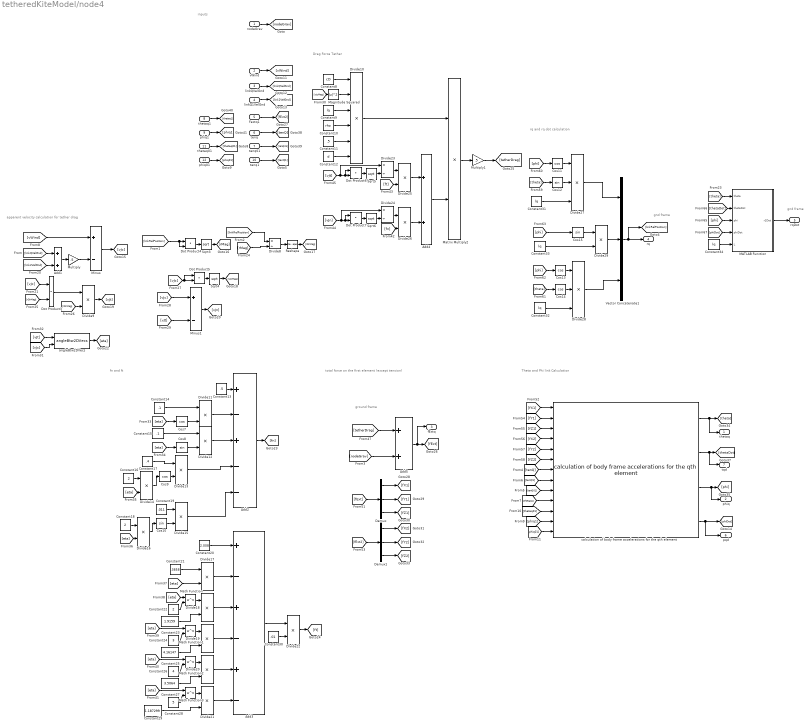
== system tetheredKiteModel/node4 ==
  note: gnd frame
  note: fn and ft
  note: gnd frame
  note: inputs
  note: apparent velocity calculation for tether drag
  note: ground frame
  note: rq and rq dot calculation
  note: Theta and Phi link Calculation
  note: total force on the first element
      |  (except tension)
  note: Drag Force Tether
  nodeGrav : Inport
  vWind : Inport  Port=2
  "linkQVelGnd " : Inport  Port=3
  linkQ1VelGnd : Inport  Port=4
  Fextq1 : Inport  Port=5
  "tenq " : Inport  Port=6
  tenq01 : Inport  Port=7
  "thetaq1 " : Inport  Port=8
  phiq1 : Inport  Port=9
  tenq1 : Inport  Port=10
  thetaq01 : Inport  Port=11
  phiq01 : Inport  Port=12
  Add1 : Sum
  Add2 : Sum  Inputs=+-+--
  Add3 : Sum  Inputs=+-+-+-
  Add4 : Sum
  Add5 : Sum
  Constant10 : Constant  Value=rho
  Constant11 : Constant  Value=.5
  Constant12 : Constant  Value=d
  Constant13 : Constant  Value=.5
  Constant14 : Constant  Value=.1
  Constant15 : Constant  Value=.1
  Constant16 : Constant  Value=2
  Constant17 : Constant  Value=.4
  Constant18 : Constant  Value=2
  Constant19 : Constant  Value=.011
  Constant20 : Constant  Value=2.008
  Constant21 : Constant  Value=.3858
  Constant22 : Constant  Value=2
  Constant23 : Constant  Value=1.9159
  Constant24 : Constant  Value=3
  Constant25 : Constant  Value=4.16147
  Constant26 : Constant  Value=4
  Constant27 : Constant  Value=3.5064
  Constant28 : Constant  Value=5
  Constant29 : Constant  Value=1.187299
  Constant30 : Constant  Value=.01
  Constant{9,31..34} (5 alike) : Constant  Value=lq
  Constant8 : Constant  Value=cD
  Cos{8,10,12,15} (4 alike) : Trigonometry
  Cos{7,9,11,13..14} (5 alike) : Trigonometry  Operator=cos
  Demux : Demux  Outputs=3
  Demux1 : Demux  Outputs=3
  Divide10 : Product  Inputs=******
  Divide{9,11..22,25..26,29} (16 alike) : Product  Inputs=**
  Divide23 : Product  Inputs=*/
  Divide24 : Product  Inputs=*/
  Divide27 : Product  Inputs=***
  Divide28 : Product  Inputs=***
  Divide8 : Product  Inputs=*/
  Dot Product{3..7} (5 alike) : DotProduct  InputSameDT=on  OutDataTypeStr=Inherit: Inherit via internal rule
  MATLAB Function : MATLAB Function  TreatAsAtomicUnit=on
  Magnitude Squared : Math  Operator=magnitude^2  SaturateOnIntegerOverflow=on
  Math Function{,1..3} (4 alike) : Math  Operator=pow  SaturateOnIntegerOverflow=on
  Matrix Multiply2 : Product
  Minus : Sum  Inputs=+-
  Minus1 : Sum  Inputs=+-
  Multiply : Gain  Gain=.5
  Multiply1 : Gain  Gain=.5
  Reshape : Reshape  OutputDimensionality=Column vector (2-D)
  Sqrt{3..6} (4 alike) : Sqrt  SaturateOnIntegerOverflow=on
  Vector Concatenate1 : Concatenate  NumInputs=3
  angleBtw2DVecs : angleBtw2Vecs_ul/angleBtw2DVecs  SystemSampleTime=-1
  calculation of body frame accelerations for the qth element : accelerationCalculator_ul/calculation of body frame accelerations for the qth element  mj=1000*200*pi*.0005*.0005  mj1=1000*200*pi*.0005*.0005  L=200
  thetaq : Outport
  phiq : Outport  Port=2
  fExtq : Outport  Port=3
  "rq " : Outport  Port=4
  rqDot : Outport  Port=5
  pqd : Outport  Port=6
  tqd : Outport  Port=7
  wires:
  Cos14/1 -> Divide28/2
  Constant32/1 -> Divide28/3
  Cos15/1 -> Divide29/1
  Constant34/1 -> MATLAB Function/5(L)
  Demux/3 -> [fZ1]
  Divide16/1 -> Cos10/1
  Cos10/1 -> Divide15/2
  Constant18/1 -> Divide16/1
  Divide21/1 -> Add3/6
  Constant21/1 -> Divide17/1
  [fZ1] -> calculation of body frame accelerations for the qth element/3
  tenq01/1 -> [tenQ01]
  [phi] -> Cos15/1
  MATLAB Function/1(r1Dot) -> rqDot/1
  [vJc] -> angleBtw2DVecs/2
  Magnitude Squared/1 -> Divide10/2
  [phi] -> Cos11/1
  [fExt] -> Demux/1
  [phiq01] -> calculation of body frame accelerations for the qth element/13
  Demux1/2 -> [fY2]
  Constant14/1 -> Divide11/1
  Demux1/1 -> [fX2]
  [eta] -> Divide17/2
  [phi] -> MATLAB Function/3(phi)
  Divide22/1 -> [ft]
  Divide15/1 -> Add2/5
  Constant11/1 -> Divide10/5
  Constant12/1 -> Divide10/6
  Divide19/1 -> Add3/4
  Cos12/1 -> Divide27/2
  [tetherDrag] -> Add5/1
  [thetaDot] -> MATLAB Function/2(thetaDot)
  [vJc] -> Dot Product5/1, Dot Product5/2
  [rMag] -> Divide8/2
  [eta] -> Cos8/1
  Constant15/1 -> Divide12/1
  Sqrt4/1 -> [vJcMag]
  Add3/1 -> Divide22/1
  Divide27/1 -> Vector Concatenate1/1
  Cos13/1 -> Divide28/1
  Sqrt3/1 -> [rMag]
  Add4/1 -> Matrix Multiply2/2
  Cos7/1 -> Divide11/2
  Multiply/1 -> Minus/2
  Vector Concatenate1/1 -> [linkRelPosition], "rq "/1
  Divide11/1 -> Add2/2
  Dot Product5/1 -> Sqrt4/1
  [vJcMag] -> Magnitude Squared/1
  Minus/1 -> [vJc]
  [theta] -> Cos14/1
  Constant33/1 -> Divide29/2
  [theta] -> MATLAB Function/1(theta)
  [rDrMag] -> Divide9/2
  Minus1/1 -> [vJn]
  Divide8/1 -> Reshape/1
  Dot Product3/1 -> Divide9/1
  [vJt] -> angleBtw2DVecs/1
  nodeGrav/1 -> [nodeGrav]
  [fX2] -> calculation of body frame accelerations for the qth element/4
  Constant23/1 -> Divide18/2
  [fY2] -> calculation of body frame accelerations for the qth element/5
  [fZ2] -> calculation of body frame accelerations for the qth element/6
  Divide29/1 -> Vector Concatenate1/2
  [vJc] -> Dot Product3/1
  Divide18/1 -> Add3/3
  [phi] -> Cos13/1
  Constant10/1 -> Divide10/4
  Constant8/1 -> Divide10/1
  [eta] -> Cos7/1
  Constant9/1 -> Divide10/3
  Divide17/1 -> Add3/2
  Dot Product4/1 -> Sqrt3/1
  Constant19/1 -> Divide15/1
  Add2/1 -> [fn]
  [vJt] -> Divide23/1, Dot Product6/1, Dot Product6/2
  Add5/1 -> fExtq/1, [fExt]
  Constant13/1 -> Add2/1
  Dot Product6/1 -> Sqrt5/1
  Constant26/1 -> Math Function2/2
  [vWind] -> Minus/1
  [vJc] -> Minus1/1
  Math Function2/1 -> Divide20/1
  [eta] -> Math Function2/1
  Constant27/1 -> Divide20/2
  Fextq1/1 -> [fExt2]
  vWind/1 -> [vWind]
  [rDrMag] -> Dot Product3/2
  [phiDot] -> MATLAB Function/4(phiDot)
  Demux/2 -> [fY1]
  Divide23/1 -> Divide25/1
  Divide26/1 -> Add4/2
  [eta] -> Divide16/2
  Constant30/1 -> Divide22/2
  Divide25/1 -> Add4/1
  Divide9/1 -> [vJt]
  Constant24/1 -> Math Function1/2
  Math Function1/1 -> Divide19/1
  Sqrt6/1 -> Divide24/2
  Demux1/3 -> [fZ2]
  Add1/1 -> Multiply/1
  [link2VelGnd] -> Add1/2
  [fX1] -> calculation of body frame accelerations for the qth element/1
  [ft] -> Divide25/2
  Constant20/1 -> Add3/1
  Divide20/1 -> Add3/5
  [thetaq1] -> calculation of body frame accelerations for the qth element/10
  "thetaq1 "/1 -> [thetaq1]
  [linkRelPosition] -> Dot Product4/2, Dot Product4/1
  [tenQ01] -> calculation of body frame accelerations for the qth element/9
  phiq1/1 -> [phiq1]
  [eta] -> Math Function3/1
  Cos8/1 -> Divide12/2
  Constant25/1 -> Divide19/2
  angleBtw2DVecs/1 -> [eta]
  Constant28/1 -> Math Function3/2
  [eta] -> Divide14/2
  Math Function3/1 -> Divide21/1
  linkQ1VelGnd/1 -> [link2VelGnd]
  Constant29/1 -> Divide21/2
  Divide24/1 -> Divide26/1
  [vJn] -> Divide24/1, Dot Product7/1, Dot Product7/2
  [tenQ] -> calculation of body frame accelerations for the qth element/7
  Constant16/1 -> Divide14/1
  Demux/1 -> [fX1]
  [eta] -> Math Function/1
  Constant17/1 -> Divide13/1
  [vJt] -> Minus1/2
  [linkRelPosition] -> Divide8/1
  Divide10/1 -> Matrix Multiply2/1
  [eta] -> Math Function1/1
  Matrix Multiply2/1 -> Multiply1/1
  Divide28/1 -> Vector Concatenate1/3
  [fY1] -> calculation of body frame accelerations for the qth element/2
  "linkQVelGnd "/1 -> [linkQVelGnd]
  [theta] -> Cos12/1
  Constant31/1 -> Divide27/3
  Sqrt5/1 -> Divide23/2
  [fn] -> Divide26/2
  Math Function/1 -> Divide18/1
  Divide13/1 -> Add2/4
  "tenq "/1 -> [tenQ]
  [nodeGrav] -> Add5/2
  Divide14/1 -> Cos9/1
  Constant22/1 -> Math Function/2
  Divide12/1 -> Add2/3
  [thetaq01] -> calculation of body frame accelerations for the qth element/11
  Multiply1/1 -> [tetherDrag]
  [tenQ1] -> calculation of body frame accelerations for the qth element/8
  Dot Product7/1 -> Sqrt6/1
  Cos11/1 -> Divide27/1
  [fExt2] -> Demux1/1
  [linkQVelGnd] -> Add1/1
  Cos9/1 -> Divide13/2
  tenq1/1 -> [tenQ1]
  thetaq01/1 -> [thetaq01]
  phiq01/1 -> [phiq01]
  [phiq1] -> calculation of body frame accelerations for the qth element/12
  Reshape/1 -> [rDrMag]
  calculation of body frame accelerations for the qth element/1 -> thetaq/1, [theta]
  calculation of body frame accelerations for the qth element/2 -> tqd/1, [thetaDot]
  calculation of body frame accelerations for the qth element/3 -> phiq/1, [phi]
  calculation of body frame accelerations for the qth element/4 -> pqd/1, [phiDot]
